simulink model "main"  (R2020b)
settings: Solver=ode23tb  StartTime=0.0  StopTime=20  FixedStep=0.0005  MaxStep=0.005  RelTol=1e-3  AbsTol=1e-3
StartFcn:
  | tic;
StopFcn:
  | Elapsed_Sim_Time = toc;
  | disp(['Elapsed Sim Time = ' num2str(Elapsed_Sim_Time)]);
model workspace (MATLAB code in the model file):
  | floor_l = 1.0900;
  | floor_d = 0.0100;
  | 
  | % PART
  | model_idx = 0;
  | model_dims = [0.06 0.06 0.06;
  |      0.02 0.05 0.07;
  |      0.04 0.04 0.10;
  |      0.05 0.05 0.05;
  |      0.10 0.08 0.08];
  | % distance between models on the conveyor belt
  | model_d = 0.12;
  | % distance to push models forwards in the -y dir (towards the box)
  | model_push = 0.2;
  | 
  | % BELT
  | belt_w = 0.1000;
  | belt_l = 1.2000;
  | belt_h = 0.0200;
  | belt_in_offset = [0 0.8000 0.0100];
  | 
  | container_belt_h = 0.02;
  | container_belt_l = 2.0;
  | container_belt_w = 0.2;
  | container_belt_offset = [-0.5050 0 -0.020];
  | 
  | belt_spd = 0.1;
  | 
  | % Model
  | cube_d = 0.06;
  | cube_z_off = belt_in_offset(3) + (container_belt_h / 2) + 0.001;
  | cube_z_offs = (model_dims(:,3) / 2) + cube_z_off;
  | 
  | % Container dimensions
  | % len, width, height are INTERNAL (Changed because most things were using internal anyway and it's 4am and we just need a working demo)
  | % Dimensions
  | container_len = 0.2;
  | container_width = 0.15;
  | container_height = 0.15;
  | container_thickness = 0.005;
  | 
  | 
  | % ????
  | cube_con_rsph = 0.003;
  | 
  | cube_con_k = 1000000;
  | cube_con_b = 1000;
  | 
  | finger_con_x = 0.01;
  | finger_con_y = 0.01;
  | finger_con_z = 5e-4;
  | finger_con_rsph = 5.0000e-04;
  | finger_con_muk = 0.05;
  | finger_con_mus = 0.07;
  | finger_con_vth = 1e-3;
  | 
  | finger_l = 0.4;
  | finger_w = 0.03;
  | finger_t = 0.01;
undefined symbols (not defined in the file): Bottom, Extr_Data_LinkHoles, Part1, Part2, Part3, Part4, Part5, point1, point2, point3, Side1, Side2, Side3, Side4, X, Y, Z
libraries: sm_lib x113, nesl_utility x35, Parts_Lib x10, Contact_Forces_Lib x6, sm_delta_robot_lib x1
(part 1 of 5)
CloseFcn:
  | try,close(h1_Gripper_2Belts),end
  | clear h1_Gripper_2Belts
  | 
  | clear simlog_Gripper_2Belts
  | clear logsout_Gripper_2Belts
Description:
  | Gripper with Conveyor Belts
  | 
  | Copyright 2017-2020 The MathWorks, Inc.
settings Model: NumberOfSteps=10000  OrderedModelArguments=off  Creator=smiller  LastModifiedBy=joeoc
settings SolverCC: AutoScaleAbsTol=off  ZcThreshold=1e-3  MaxConsecutiveZCs=500
settings DataIOCC: MaxDataPoints=15000  SignalLoggingName=logsout_Gripper_2Belts
settings OptimizationCC: SimCompilerOptimization=on
settings DebuggingCC: ReadBeforeWriteMsg=DisableAll  WriteAfterWriteMsg=DisableAll  WriteAfterReadMsg=DisableAll  MultiTaskDSMMsg=none  ModelReferenceExtraNoncontSigs=warning  PregeneratedLibrarySubsystemCodeDiagnostic=none  ArithmeticOperatorsInVariantConditions=warning
settings ModelReferenceCC: UpdateModelReferenceTargets=IfOutOfDate
settings SFSimCC: SimCustomHeaderCode="#include \"src/process_optimiser.h\""  SimUserSources=src/process_optimiser.cc  SFSimEcho=off  SimUseLocalCustomCode=off  CustomCodeUndefinedFunction=ThrowError  SimTargetLang=C++
settings RTWCC: RTWUseLocalCustomCode=off  BuildConfiguration=Faster Runs
settings CodeAppCC: StateflowObjectComments=on
settings SimscapeCC: SimscapeNormalizeSystem=off  SimscapeLogType=all  SimscapeLogSimulationStatistics=on  SimscapeLogToSDI=on  SimscapeLogOpenViewer=on  SimscapeLogName=simlog_consignment_tetris  SimscapeLogDecimation=2  SimscapeLogDataHistory=20000
settings DiagnosticsConfigSet: SimMechanicsRigidlyBoundBlock=none
settings ExplorerConfigSet: InternalSimMechanicsExplorerSettings="<ExplorerConfiguration><canonicalview>default</canonicalview><AnimationSetting><BasePlaybackSpeed>1.0</BasePlaybackSpeed><PlaybackSpeedFactor>0.03125</PlaybackSpeedFactor></AnimationSetting><TilePanel><TileInfo><Tiles Columns=\"2\" Count=\"3\" Rows=\"2\"><Column Weight=\"0.7465\"/><Column Weight=\"0.2535\"/><Row Weight=\"0.4991\"/><Row Weight=\"0.5009\"/><Tile Height=\"2\" Width=\"1\" X=\"0\" Y=\"0\"/><Tile Height=\"1\" Width=\"1\" X=\"1\" Y=\"0\"/><Tile Height=\"1\" Width=\"1\" X=\"1\" Y=\"1\"/></Tiles></TileInfo><SceneInfo><SceneViewer><BGColor><R>0.800000011920928955</R><G>1</G><B>1</B></BGColor><Camera><DoPerspective>off</DoPerspective><Position><X>-1.30631954778313775</X><Y>0.698143211261454399</Y><Z>1.90762010333630316</Z></Position><Center><X>-0.281765838627846099</X><Y>0.411252835223805402</Y><Z>0.511382897183640939</Z></Center><Up><X>0.749738551919228224</X><Y>-0.267711821281975237</Y><Z>0.605163188331830471</Z></Up><ViewLimDist>1</ViewLimDist><YLim>0.375389099339456467</YLim><XLim>0.530237102816982331</XLim></Camera></SceneViewer><SceneViewer><BGColor><R>0.800000011920928955</R><G>1</G><B>1</B></BGColor><Camera><DoPerspective>off</DoPerspective><Position><X>-1.84239040145380972</X><Y>0.117407489698812761</Y><Z>0.195367996009015804</Z></Position><Center><X>-0.504999962495096044</X><Y>0.117407489698812761</Y><Z>0.195367996009015804</Z></Center><Up><X>0</X><Y>0</Y><Z>1</Z></Up><ViewLimDist>1</ViewLimDist><YLim>0.230836944692208057</YLim><XLim>0.223282281047735787</XLim></Camera></SceneViewer><SceneViewer><BGColor><R>0.800000011920928955</R><G>1</G><B>1</B></BGColor><Camera><DoPerspective>on</DoPerspective><Position><X>1.1754095475261223e-18</X><Y>-8.63362207815730793e-18</Y><Z>0.640000000000000013</Z></Position><Center><X>2.95506551950155109e-05</X><Y>0.202260727586032307</Y><Z>0.110212737904600094</Z></Center><Up><X>1</X><Y>1.11473304577392036e-30</Y><Z>-2.39270069167019591e-15</Z></Up><ViewLimDist>1</ViewLimDist><YLim>0.466307658154998583</YLim><XLim>0.449412453149382662</XLim></Camera></SceneViewer></SceneInfo></TilePanel><MechEditorPanel><Cameras><Camera><Id>Camera1</Id><Value><Name>TopCamera</Name><NativeCamera><PositionTrackingFeature>Delta_Robot.Camera_Frame</PositionTrackingFeature><CenterTrackingFeature>Delta_Robot.End_Effector_Frame</CenterTrackingFeature><UpVectorTrackingFeature>Delta_Robot.End_Effector_Frame</UpVectorTrackingFeature><CenterTrackingOrigin>on</CenterTrackingOrigin><UpVectorTrackingDirection>+X</UpVectorTrackingDirection></NativeCamera></Value></Camera></Cameras><GfxPanelCameraMap><MapElement CameraMLId=\"Camera1\" GfxPanelIndex=\"2\"/></GfxPanelCameraMap><VideoCreator><PlaybackSpeedRatio>0.25</PlaybackSpeedRatio><FrameRate>60</FrameRate><VideoFormat>MPEG-4</VideoFormat><FrameSize>[1280 720]</FrameSize></VideoCreator></MechEditorPanel></ExplorerConfiguration>"

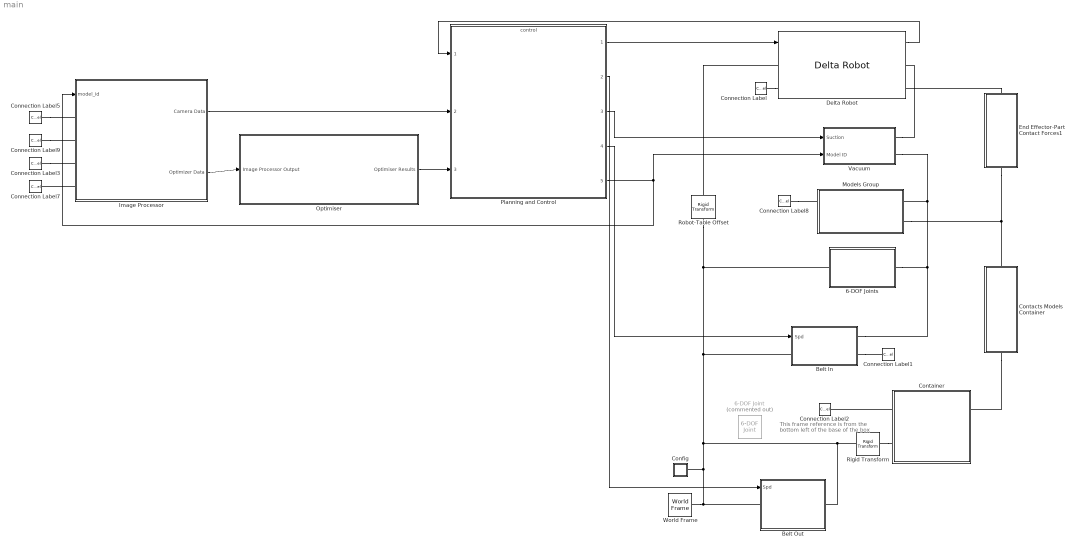
== system main ==
  note: This frame reference is from the bottom left of the base of the box
  6-DOF Joint : sm_lib/Joints/6-DOF Joint  Commented=on  JointMode=Normal  SenseConstraintForce=off  SenseConstraintForceX=off  SenseConstraintForceY=off  SenseConstraintForceZ=off  SenseConstraintTorque=off  SenseConstraintTorqueX=off  SenseConstraintTorqueY=off  SenseConstraintTorqueZ=off  SenseTotalForce=off  SenseTotalForceX=off  SenseTotalForceY=off  SenseTotalForceZ=off  SenseTotalTorque=off  SenseTotalTorqueX=off  SenseTotalTorqueY=off  SenseTotalTorqueZ=off  CompositeWrenchDir=FollowerOnBase  CompositeWrenchFrame=BaseFrame  PxEquilibriumPosition=0  PxEquilibriumPositionUnits=m  PxSpringStiffness=0  PxSpringStiffnessUnits=N/m  PxDampingCoefficient=0  PxDampingCoefficientUnits=N/(m/s)  PxTorqueActuationMode=NoTorque  PxMotionActuationMode=ComputedMotion  PxSensePosition=off  PxSenseVelocity=off  PxSenseAcceleration=off  PxSenseTorqueForce=off  PxSenseLowerLimitTorqueForce=off  PxSenseUpperLimitTorqueForce=off  PxLowerLimitSpecify=off  PxLowerLimitBound=-1  PxLowerLimitBoundUnits=m  PxLowerLimitStiffness=1e6  PxLowerLimitStiffnessUnits=N/m  PxLowerLimitDamping=1e3  PxLowerLimitDampingUnits=N/(m/s)  PxLowerLimitTransitionRegionWidth=1e-4  PxLowerLimitTransitionRegionWidthUnits=m  PxUpperLimitSpecify=off  PxUpperLimitBound=1  PxUpperLimitBoundUnits=m  PxUpperLimitStiffness=1e6  PxUpperLimitStiffnessUnits=N/m  PxUpperLimitDamping=1e3  PxUpperLimitDampingUnits=N/(m/s)  PxUpperLimitTransitionRegionWidth=1e-4  PxUpperLimitTransitionRegionWidthUnits=m  PxPositionTargetSpecify=off  PxPositionTargetPriority=High  PxPositionTargetValue=0  PxPositionTargetValueUnits=m  PxVelocityTargetSpecify=off  PxVelocityTargetPriority=High  PxVelocityTargetValue=0  PxVelocityTargetValueUnits=m/s  PyEquilibriumPosition=0  PyEquilibriumPositionUnits=m  PySpringStiffness=0  PySpringStiffnessUnits=N/m  PyDampingCoefficient=0  PyDampingCoefficientUnits=N/(m/s)  PyTorqueActuationMode=NoTorque  PyMotionActuationMode=ComputedMotion  PySensePosition=off  PySenseVelocity=off  PySenseAcceleration=off  PySenseTorqueForce=off  PySenseLowerLimitTorqueForce=off  PySenseUpperLimitTorqueForce=off  PyLowerLimitSpecify=off  PyLowerLimitBound=-1  PyLowerLimitBoundUnits=m  PyLowerLimitStiffness=1e6  PyLowerLimitStiffnessUnits=N/m  PyLowerLimitDamping=1e3  PyLowerLimitDampingUnits=N/(m/s)  PyLowerLimitTransitionRegionWidth=1e-4  PyLowerLimitTransitionRegionWidthUnits=m  PyUpperLimitSpecify=off  PyUpperLimitBound=1  PyUpperLimitBoundUnits=m  PyUpperLimitStiffness=1e6  PyUpperLimitStiffnessUnits=N/m  PyUpperLimitDamping=1e3  PyUpperLimitDampingUnits=N/(m/s)  PyUpperLimitTransitionRegionWidth=1e-4  PyUpperLimitTransitionRegionWidthUnits=m  PyPositionTargetSpecify=off  PyPositionTargetPriority=High  PyPositionTargetValue=0  PyPositionTargetValueUnits=m  PyVelocityTargetSpecify=off  PyVelocityTargetPriority=High  PyVelocityTargetValue=0  PyVelocityTargetValueUnits=m/s  PzEquilibriumPosition=0  PzEquilibriumPositionUnits=m  PzSpringStiffness=0  PzSpringStiffnessUnits=N/m  PzDampingCoefficient=0  PzDampingCoefficientUnits=N/(m/s)  PzTorqueActuationMode=NoTorque  PzMotionActuationMode=ComputedMotion  PzSensePosition=off  PzSenseVelocity=off  PzSenseAcceleration=off  PzSenseTorqueForce=off  PzSenseLowerLimitTorqueForce=off  PzSenseUpperLimitTorqueForce=off  PzLowerLimitSpecify=off  PzLowerLimitBound=-1  PzLowerLimitBoundUnits=m  PzLowerLimitStiffness=1e6  PzLowerLimitStiffnessUnits=N/m  PzLowerLimitDamping=1e3  PzLowerLimitDampingUnits=N/(m/s)  PzLowerLimitTransitionRegionWidth=1e-4  PzLowerLimitTransitionRegionWidthUnits=m  PzUpperLimitSpecify=off  PzUpperLimitBound=1  PzUpperLimitBoundUnits=m  PzUpperLimitStiffness=1e6  PzUpperLimitStiffnessUnits=N/m  PzUpperLimitDamping=1e3  PzUpperLimitDampingUnits=N/(m/s)  PzUpperLimitTransitionRegionWidth=1e-4  PzUpperLimitTransitionRegionWidthUnits=m  PzPositionTargetSpecify=off  PzPositionTargetPriority=High  PzPositionTargetValue=0  PzPositionTargetValueUnits=m  PzVelocityTargetSpecify=off  PzVelocityTargetPriority=High  PzVelocityTargetValue=0  PzVelocityTargetValueUnits=m/s  SphDefPosRotationMethod=None  SphDefPosRotationAngleUnits=deg  SphDefPosRotationStandardAxis=+Z  SphDefPosRotationAngle=0.0  SphDefPosRotationArbitraryAxis=[0 0 1]  SphDefPosFollAlignAxisA=+X  SphDefPosBaseAlignAxisA=+Y  SphDefPosFollAlignAxisB=+Y  SphDefPosBaseAlignAxisB=+Z  SphDefPosRotationSequenceAxes=FollowerAxes  SphDefPosRotationSequence=XYX  SphDefPosRotationSequenceAngles=[0 0 0]  SphDefPosRotationSequenceAnglesUnits=deg  SphDefPosRotationMatrix=[1 0 0; 0 1 0; 0 0 1]  SphEqPosRotationMethod=None  SphEqPosRotationAngleUnits=deg  SphEqPosRotationStandardAxis=+Z  SphEqPosRotationAngle=0.0  SphEqPosRotationArbitraryAxis=[0 0 1]  SphEqPosFollAlignAxisA=+X  SphEqPosBaseAlignAxisA=+Y  SphEqPosFollAlignAxisB=+Y  SphEqPosBaseAlignAxisB=+Z  SphEqPosRotationSequenceAxes=FollowerAxes  SphEqPosRotationSequence=XYX  SphEqPosRotationSequenceAngles=[0 0 0]  SphEqPosRotationSequenceAnglesUnits=deg  SphEqPosRotationMatrix=[1 0 0; 0 1 0; 0 0 1]  SphSpringStiffness=0  SphSpringStiffnessUnits=N*m/deg  SphDampingCoefficient=0  SphDampingCoefficientUnits=N*m/(deg/s)  SphActuateTorqueX=off  SphActuateTorqueY=off  SphActuateTorqueZ=off  SphActuateTorque=off  SphTorqueActuationMode=NoTorque  SphMotionActuationMode=ComputedMotion  SphActuationFrame=BaseFrame  SphSensePosition=off  SphSenseVelocityX=off  SphSenseVelocityY=off  SphSenseVelocityZ=off  SphSenseVelocity=off  SphSenseAccelerationX=off  SphSenseAccelerationY=off  SphSenseAccelerationZ=off  SphSenseAcceleration=off  SphSenseTorqueX=off  SphSenseTorqueY=off  SphSenseTorqueZ=off  SphSenseTorqueForce=off  SphSenseLowerLimitTorqueMag=off  SphSenseUpperLimitTorqueMag=off  SphSensingFrame=BaseFrame  SphLowerLimitSpecify=off  SphLowerLimitBound=15  SphLowerLimitBoundUnits=deg  SphLowerLimitStiffness=1e4  SphLowerLimitStiffnessUnits=N*m/deg  SphLowerLimitDamping=10  SphLowerLimitDampingUnits=N*m/(deg/s)  SphLowerLimitTransitionRegionWidth=0.1  SphLowerLimitTransitionRegionWidthUnits=deg  SphUpperLimitSpecify=off  SphUpperLimitBound=45  SphUpperLimitBoundUnits=deg  SphUpperLimitStiffness=1e4  SphUpperLimitStiffnessUnits=N*m/deg  SphUpperLimitDamping=10  SphUpperLimitDampingUnits=N*m/(deg/s)  SphUpperLimitTransitionRegionWidth=0.1  SphUpperLimitTransitionRegionWidthUnits=deg  SphPositionTargetRotationMethod=None  SphPositionTargetRotationAngleUnits=deg  SphPositionTargetRotationStandardAxis=+Z  SphPositionTargetRotationAngle=0.0  SphPositionTargetRotationArbitraryAxis=[0 0 1]  SphPositionTargetFollAlignAxisA=+X  SphPositionTargetBaseAlignAxisA=+Y  SphPositionTargetFollAlignAxisB=+Y  SphPositionTargetBaseAlignAxisB=+Z  SphPositionTargetRotationSequenceAxes=FollowerAxes  SphPositionTargetRotationSequence=XYX  SphPositionTargetRotationSequenceAngles=[0 0 0]  SphPositionTargetRotationSequenceAnglesUnits=deg  SphPositionTargetRotationMatrix=[1 0 0; 0 1 0; 0 0 1]  SphPositionTargetSpecify=off  SphPositionTargetPriority=High  SphVelocityTargetValue=[0 0 0]  SphVelocityTargetValueUnits=deg/s  SphVelocityTargetSpecify=off  SphVelocityTargetPriority=High  SphVelocityTargetInFollowerFrame=on
  6-DOF Joints : Subsystem
  Belt In : Subsystem  mask{stff=1e3, dmp=1.4e2}
      mask prompts: stff "Stiffness"; dmp "Damping"
      mask Display: image('$imagefile'); % Use "Edit Image" on toolstrip to change.
  Belt Out : Subsystem  mask{stff=5e2, dmp=1.4e1}
      mask prompts: stff "Stiffness"; dmp "Damping"
      mask Display: image('$imagefile'); % Use "Edit Image" on toolstrip to change.
  Config : Subsystem
  Connection Label : ConnectionLabel  Label=Camera
  Connection Label1 : ConnectionLabel  Label=Belt_In_End
  Connection Label2 : ConnectionLabel  Label=Container
  Connection Label3 : ConnectionLabel  Label=Container
  Connection Label5 : ConnectionLabel  Label=Camera
  Connection Label7 : ConnectionLabel  Label=Belt_In_End
  Connection Label8 : ConnectionLabel  Label=Parts
  Connection Label9 : ConnectionLabel  Label=Parts
  Contacts Models Container : Subsystem  mask{k=500, b=10, mus=0.4, muk=0.4}
      mask prompts: k "Stiffness (N/m)"; b "Dampink (N/(m/s))"; mus "Coefficient of Static Friction"; muk "Coefficient of Dynamic Friction"
      mask DialogControl Control2 Prompt: Force Parameters
  Container : Subsystem  Tag=CustomStyle  mask{box_l=container_len, box_w=container_width, box_h=container_height, box_wt=container_thickness, box_opacity=1.0, box_color=[0.8 0.5 0.11]}
      mask prompts: box_l "Length (m)"; box_w "Width (m)"; box_h "Height (m)"; box_wt "Wall thickness (m)"; box_opacity "Opacity"; box_color "Color"
      mask init:
      | x = [[1 1 -1 -1 1]*(box_l/2+box_wt) [1 -1 -1 1 1]*box_l/2];
      | y = [[1 -1 -1 1 1]*(box_w/2+box_wt) [1 1 -1 -1 1]*box_w/2];
      | box_extr = flipud([x' y']);
      mask DialogControl Control2 Prompt: Box Dimensions
      mask Display: image('$imagefile'); % Use "Edit Image" on toolstrip to change.
  Delta Robot : sm_delta_robot_lib/Delta Robot  Rtop=0.15  Rbot=0.03  L1=0.2  R1=0.01  L2=0.5  L3=0.07  R2=0.005  eeL=0.03  eeR=0.01  th0=[10; 10; 10]  thd0=[0 0 0]  mask(Delta Robot){}
      mask init:
      | clear delta_robot_kf delta_robot_ik
      settings: SourceProductBaseCode=MS
  End Effector-Part Contact Forces1 : Subsystem  mask(End Effector-Part Contact Forces){k=1e5, b=100, mus=0.6, muk=0.6}
      mask prompts: k "Stiffness (N/m)"; b "Damping (N/(m/s))"; mus "Coefficient of Static Friction"; muk "Coefficient of Dynamic Friction"
      mask help: This block models the contact forces between the end effector and the part. The entire cylindrical part geometry is used, but the end effector geometry corresponds to the three contact points around the tip.
  Image Processor : Subsystem
      mask Display: image('$imagefile'); % Use "Edit Image" on toolstrip to change.
  Models Group : Subsystem  Tag=CustomStyle
      mask Display: image('$imagefile'); % Use "Edit Image" on toolstrip to change.
  Optimiser : Subsystem
  Planning and Control : ModelReference  ModelNameDialog=control.slx  SimulationMode=Normal  ModelReferenceVersion=1.112
  Rigid Transform : sm_lib/Frames and Transforms/Rigid Transform  TranslationMethod=StandardAxis  TranslationStandardOffset=container_thickness * 1.5  TranslationLengthUnit=m  TranslationStandardAxis=-Z  TranslationCartesianOffset=[0 0 0]  TranslationROffset=0  TranslationROffsetUnits=m  TranslationZOffset=0  TranslationZOffsetUnits=m  TranslationThetaOffset=0  TranslationThetaOffsetUnits=deg  RotationMethod=None  RotationAngleUnits=deg  RotationStandardAxis=+Z  RotationAngle=0.0  RotationArbitraryAxis=[0 0 1]  FollAlignAxisA=+X  BaseAlignAxisA=+Y  FollAlignAxisB=+Y  BaseAlignAxisB=+Z  RotationSequenceAxes=FollowerAxes  RotationSequence=XYX  RotationSequenceAngles=[0 0 0]  RotationSequenceAnglesUnits=deg  RotationMatrix=[1 0 0; 0 1 0; 0 0 1]
  Robot-Table Offset : sm_lib/Frames and Transforms/Rigid Transform  TranslationMethod=StandardAxis  TranslationStandardOffset=0.65  TranslationLengthUnit=m  TranslationStandardAxis=+Z  TranslationCartesianOffset=[0 0 0]  TranslationROffset=0  TranslationROffsetUnits=m  TranslationZOffset=0  TranslationZOffsetUnits=m  TranslationThetaOffset=0  TranslationThetaOffsetUnits=deg  RotationMethod=None  RotationAngleUnits=deg  RotationStandardAxis=+Z  RotationAngle=0.0  RotationArbitraryAxis=[0 0 1]  FollAlignAxisA=+Z  BaseAlignAxisA=-Z  FollAlignAxisB=+X  BaseAlignAxisB=+X  RotationSequenceAxes=FollowerAxes  RotationSequence=XYX  RotationSequenceAngles=[0 0 0]  RotationSequenceAnglesUnits=deg  RotationMatrix=[1 0 0; 0 1 0; 0 0 1]
      settings: SourceProductName=Multibody
  Vacuum : Subsystem  mask(Vacuum){F=200}
      mask prompts: F "Suction Force (N)"
      mask help: This block models a simple vacuum force in which equal and opposite constant forces are applied to two frames along the line connecting their origins. The force is only applied when the Suction signal is true.
  World Frame : sm_lib/Frames and Transforms/World Frame
  wires:
  Planning and Control/1 -> Delta Robot/1
  Delta Robot/1 -> Planning and Control/1
  Image Processor/2(Optimizer Data) -> Optimiser/1(Image Processor Output)
  Planning and Control/5 -> Vacuum/2(Model ID), Image Processor/1(model_id)
  Optimiser/1(Optimiser Results) -> Planning and Control/3
  Image Processor/1(Camera Data) -> Planning and Control/2
  Planning and Control/3 -> Vacuum/1(Suction)
  Planning and Control/4 -> Belt In/1(Spd)
  Planning and Control/2 -> Belt Out/1(Spd)
  connections:
  Delta Robot/RConn2 -- End Effector-Part Contact Forces1/LConn1
  Vacuum/RConn1 -- Delta Robot/RConn1
  Delta Robot/LConn1 -- Robot-Table Offset/RConn1
  Contacts Models Container/LConn1 -- Container/RConn1
  Rigid Transform/LConn1 -- Belt Out/RConn1 -- Belt In/LConn1 -- Robot-Table Offset/LConn1 -- 6-DOF Joints/LConn1 -- Belt Out/LConn1 -- World Frame/RConn1 -- Config/RConn1
  Connection Label5/LConn1 -- Image Processor/LConn1
  Connection Label/LConn1 -- Delta Robot/LConn2
  Container/LConn1 -- Connection Label2/LConn1
  Image Processor/LConn4 -- Connection Label7/LConn1
  Models Group/RConn2 -- End Effector-Part Contact Forces1/RConn1 -- Contacts Models Container/RConn1
  Connection Label9/LConn1 -- Image Processor/LConn2
  Connection Label3/LConn1 -- Image Processor/LConn3
  Vacuum/RConn2 -- Belt In/RConn1 -- 6-DOF Joints/RConn1 -- Models Group/RConn1
  Connection Label8/LConn1 -- Models Group/LConn1
  Belt In/RConn2 -- Connection Label1/LConn1
  Rigid Transform/RConn1 -- Container/LConn2
